simulink model "regionprop_test"  (R2015b)
settings: Solver=VariableStepAuto  StartTime=0.0  StopTime=inf  RelTol=1e-3
PreLoadFcn:
  | coeff = load(coeff_save.mat);
values from neighbouring files (symbols this model uses):
  D = img(max(r2+(c2-1)*sx,1))    [IntegralImage_BoxIntegral_mine.m]
undefined symbols (not defined in the file or in its folder): IsPositionTracked, IsSkeletonTracked, JointDepthIndices, JointImageIndices, JointTrackingState, JointWorldCoordinates, PositionDepthIndices, PositionImageIndices, PositionWorldCoordinates, SegmentationData, SkeletonTrackingID, videoinput
libraries: neural x20, visionsinks x3, visionstatistics x1, imaqlib x1, visionsources x1
(part 1 of 3)
settings Model: Creator=FLM  LastModifiedBy=User

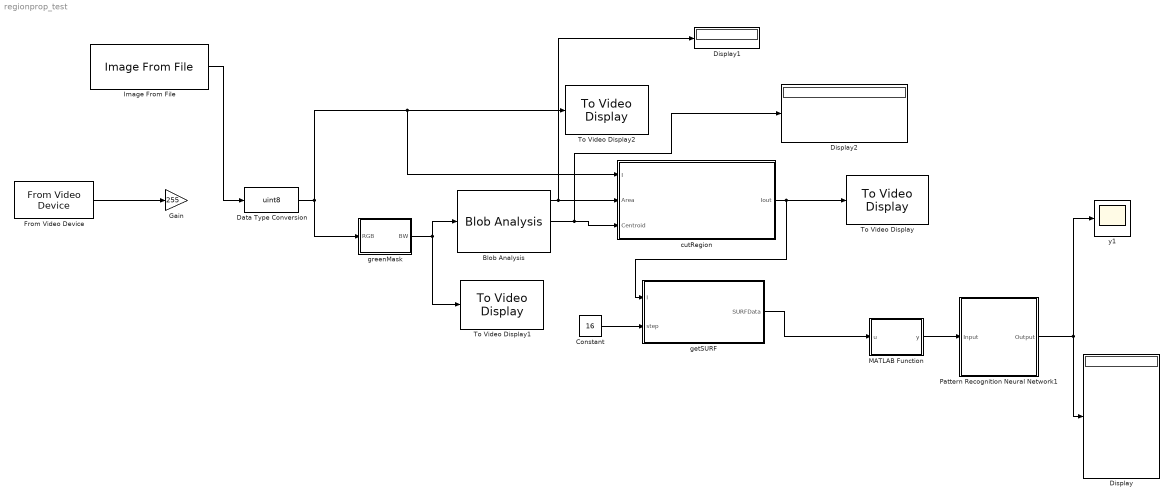
== system regionprop_test ==
  Blob Analysis : visionstatistics/Blob Analysis  Tag=vipblks_row_conv  area=on  centroid=on  bBox=on  majorAxis=off  minorAxis=off  angle=off  eccentricity=off  equivDiameterSq=off  extent=off  perimeter=off  maxBlobs=10  warnIfNumBlobsExceeded=on  isCount=off  useMinArea=off  minArea=0  useMaxArea=off  maxArea=intmax('uint32')  excludeBorderBlob=off  outDT=double  isOutVarDim=off  isFill=on  fillValues=-1  conn=8  isLabel=off  outputMode=Binary point scaling  outputWordLength=32  outputFracLength=16  firstCoeffMode=Binary point scaling  firstCoeffWordLength=16  firstCoeffFracLength=14  secondCoeffMode=Binary point scaling  secondCoeffWordLength=32  secondCoeffFracLength=16  accumMode=Binary point scaling  accumWordLength=32  accumFracLength=0  prodOutputMode=Binary point scaling  prodOutputWordLength=32  prodOutputFracLength=16  roundingMode=Floor  overflowMode=off
  Constant : Constant  Value=16
  Data Type Conversion : DataTypeConversion  OutDataTypeStr=uint8
  Display : Display
  Display1 : Display
  Display2 : Display
  From Video Device : imaqlib/From Video Device  DeviceMenu=winvideo 1 (1.3M HD WebCam)  Device=winvideo 1 (Microsoft? LifeCam Cinema(TM))  ObjConstructor=videoinput('winvideo', 1)  VideoFormatMenu=MJPG_1280x800  VideoFormat=MJPG_320x240  VideoSource=input1  ROIPosition=[0 0 240 320]  EnableHWTrigger=off  TriggerConfiguration=winvideo 1 (1.3M HD WebCam)  SampleTime=1/30  OutputPortsMode=One multidimensional signal  DataType=single  CanDoHWTrigger=no  ReturnedColorSpace=rgb  BlockHandle=1970.0024  ROIWidth=320  ROIHeight=240  ROIColumn=0  ROIRow=0  EngXMLPath=D:\Program Files\MATLAB\R2015b\toolbox\imaq\imaq\private  DevXMLPath=D:\MATLAB\SupportPackages\R2015b\osgenericvideointerface\toolbox\imaq\supportpackages\genericvideo\adaptor\win64  EngLibPath=D:\Program Files\MATLAB\R2015b\toolbox\imaq\imaqblks\imaqmex\win64  ColorSpace=rgb  BayerSensorAlignment=grbg  AllMetadata=IsPositionTracked;IsSkeletonTracked;JointDepthIndices;JointImageIndices;JointTrackingState;JointWorldCoordinates;PositionDepthIndices;PositionImageIndices;PositionWorldCoordinates;SegmentationData;SkeletonTrackingID
  Gain : Gain  Gain=255
  Image From File : visionsources/Image From File  Tag=vipblks_nd  FileName=C:\Users\User\Documents\Ponts 2015-2016\Projet dpt\github\Robot-Sur-Mars\BiggerObjects\Glue\Glue1.png  imagePorts=One multidimensional signal  Ts=inf  ImageDataType=Inherit from input image  Signed=on  WordLength=16  sdImageDataType=uint(8)  FractionLengthMode=User-defined  FractionLength=15  OutPortLabels=R|G|B
  MATLAB Function : MATLAB Function  TreatAsAtomicUnit=on
  Pattern Recognition Neural Network1 : Subsystem
      mask help: Pattern Recognition Neural Network
      mask Display: e = 0.06;c1 = [120 150 230]/255;c2 = ([120 150 230]+0)/383;c3 = ([120 150 230]+128)/383;patch([0 1 1 0],[0 0 1 1],c1);patch([0 1 1 1-e 1-e 0+e],[0 0 1 1-e 0+e 0+e],c2);patch([0 0 1 1-e 0+e 0+e],[0 1 1 1-e 1-e 0+e],c3);plot([0 1 1 0 0],[0 0 1 1 0]);fprintf('NNET');port_label('input',1,' Input');port_label('output',1,'Output ');
  To Video Display : visionsinks/To Video Display  windowSizeMode=Normal  openAtMdlStart=on  fullScreen=off  videoWindowX=1478  videoWindowY=273  saveWindowSize=off  videoWindowWidth=160  videoWindowHeight=160  inputColorFormat=RGB  inputType=Obsolete  imagePorts=One multidimensional signal  OutputDevice=On-screen video monitor  dataOrg=Column-major  isWindowOpen=off
  To Video Display1 : visionsinks/To Video Display  windowSizeMode=Normal  openAtMdlStart=on  fullScreen=off  videoWindowX=839  videoWindowY=303  saveWindowSize=off  videoWindowWidth=160  videoWindowHeight=160  inputColorFormat=RGB  inputType=Obsolete  imagePorts=One multidimensional signal  OutputDevice=On-screen video monitor  dataOrg=Column-major  isWindowOpen=off
  To Video Display2 : visionsinks/To Video Display  windowSizeMode=Normal  openAtMdlStart=on  fullScreen=off  videoWindowX=1504  videoWindowY=564  saveWindowSize=off  videoWindowWidth=160  videoWindowHeight=160  inputColorFormat=RGB  inputType=Obsolete  imagePorts=One multidimensional signal  OutputDevice=On-screen video monitor  dataOrg=Column-major  isWindowOpen=off
  cutRegion : MATLAB Function  TreatAsAtomicUnit=on
  getSURF : MATLAB Function  TreatAsAtomicUnit=on
  greenMask : MATLAB Function  TreatAsAtomicUnit=on
  y1 : Scope
      mask Display: e = 0.06;c1 = [120 230 180]/255;c2 = ([120 230 180]+0)/(256+128);c3 = ([120 230 180]+128)/(256+128);patch([0 1 1 0],[0 0 1 1],c1);patch([0 1 1 1-e 1-e 0+e],[0 0 1 1-e 0+e 0+e],c2);patch([0 0 1 1-e 0+e 0+e],[0 1 1 1-e 1-e 0+e],c3);plot([0 1 1 0 0],[0 0 1 1 0]);plot([0.15 0.85 0.85 0.15 0.15],[0.5 0.5 0.85 0.85 0.5]);
  wires:
  greenMask/1(BW) -> Blob Analysis/1, To Video Display1/1
  Blob Analysis/2 -> Display2/1, cutRegion/3(Centroid)
  Blob Analysis/1 -> cutRegion/2(Area), Display1/1
  Constant/1 -> getSURF/2(step)
  cutRegion/1(Iout) -> To Video Display/1, getSURF/1(I)
  From Video Device/1 -> Gain/1
  Data Type Conversion/1 -> cutRegion/1(I), To Video Display2/1, greenMask/1(RGB)
  getSURF/1(SURFData) -> MATLAB Function/1(u)
  MATLAB Function/1(y) -> Pattern Recognition Neural Network1/1(Input)
  Image From File/1 -> Data Type Conversion/1
  Pattern Recognition Neural Network1/1(Output) -> Display/1, y1/1

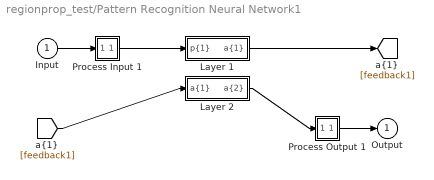
== system regionprop_test/Pattern Recognition Neural Network1 ==
  Input : Inport  PortDimensions=349
      mask Display: e = 0.06;c1 = [120 230 180]/255;c2 = ([120 230 180]+0)/(256+128);c3 = ([120 230 180]+128)/(256+128);patch([0 1 1 0],[0 0 1 1],c1);patch([0 1 1 1-e 1-e 0+e],[0 0 1 1-e 0+e 0+e],c2);patch([0 0 1 1-e 0+e 0+e],[0 1 1 1-e 1-e 0+e],c3);plot([0 1 1 0 0],[0 0 1 1 0]);
  Layer 1 : Subsystem
      mask Display: e = 0.06;c1 = [120 150 230]/255;c2 = ([120 150 230]+0)/383;c3 = ([120 150 230]+128)/383;patch([0 1 1 0],[0 0 1 1],c1);patch([0 1 1 1-e 1-e 0+e],[0 0 1 1-e 0+e 0+e],c2);patch([0 0 1 1-e 0+e 0+e],[0 1 1 1-e 1-e 0+e],c3);plot([0 1 1 0 0],[0 0 1 1 0]);
  Layer 2 : Subsystem
      mask Display: e = 0.06;c1 = [120 150 230]/255;c2 = ([120 150 230]+0)/383;c3 = ([120 150 230]+128)/383;patch([0 1 1 0],[0 0 1 1],c1);patch([0 1 1 1-e 1-e 0+e],[0 0 1 1-e 0+e 0+e],c2);patch([0 0 1 1-e 0+e 0+e],[0 1 1 1-e 1-e 0+e],c3);plot([0 1 1 0 0],[0 0 1 1 0]);
  Process Input 1 : Subsystem
      mask Display: e = 0.06;c1 = [120 150 230]/255;c2 = ([120 150 230]+0)/383;c3 = ([120 150 230]+128)/383;patch([0 1 1 0],[0 0 1 1],c1);patch([0 1 1 1-e 1-e 0+e],[0 0 1 1-e 0+e 0+e],c2);patch([0 0 1 1-e 0+e 0+e],[0 1 1 1-e 1-e 0+e],c3);plot([0 1 1 0 0],[0 0 1 1 0]);
  Process Output 1 : Subsystem
      mask Display: e = 0.06;c1 = [120 150 230]/255;c2 = ([120 150 230]+0)/383;c3 = ([120 150 230]+128)/383;patch([0 1 1 0],[0 0 1 1],c1);patch([0 1 1 1-e 1-e 0+e],[0 0 1 1-e 0+e 0+e],c2);patch([0 0 1 1-e 0+e 0+e],[0 1 1 1-e 1-e 0+e],c3);plot([0 1 1 0 0],[0 0 1 1 0]);
  Output : Outport  InitialOutput=[0;0;0;0;0;0;0]
      mask Display: e = 0.06;c1 = [120 230 180]/255;c2 = ([120 230 180]+0)/(256+128);c3 = ([120 230 180]+128)/(256+128);patch([0 1 1 0],[0 0 1 1],c1);patch([0 1 1 1-e 1-e 0+e],[0 0 1 1-e 0+e 0+e],c2);patch([0 0 1 1-e 0+e 0+e],[0 1 1 1-e 1-e 0+e],c3);plot([0 1 1 0 0],[0 0 1 1 0]);
  wires:
  Input/1 -> Process Input 1/1(x)
  Process Output 1/1(y) -> Output/1
  Process Input 1/1(p) -> Layer 1/1("p{1}")
  Layer 1/1("a{1}") -> [feedback1]
  [feedback1] -> Layer 2/1("a{1} ")
  Layer 2/1("a{2}") -> Process Output 1/1(a)

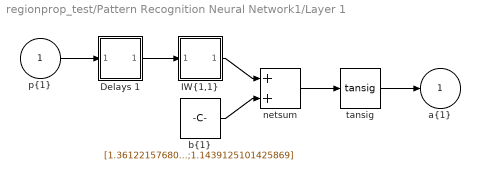
== system regionprop_test/Pattern Recognition Neural Network1/Layer 1 ==
  "p{1}" : Inport  PortDimensions=349
      mask Display: e = 0.06;c1 = [120 230 180]/255;c2 = ([120 230 180]+0)/(256+128);c3 = ([120 230 180]+128)/(256+128);patch([0 1 1 0],[0 0 1 1],c1);patch([0 1 1 1-e 1-e 0+e],[0 0 1 1-e 0+e 0+e],c2);patch([0 0 1 1-e 0+e 0+e],[0 1 1 1-e 1-e 0+e],c3);plot([0 1 1 0 0],[0 0 1 1 0]);
  Delays 1 : Subsystem
      mask Display: e = 0.06;c1 = [120 150 230]/255;c2 = ([120 150 230]+0)/383;c3 = ([120 150 230]+128)/383;patch([0 1 1 0],[0 0 1 1],c1);patch([0 1 1 1-e 1-e 0+e],[0 0 1 1-e 0+e 0+e],c2);patch([0 0 1 1-e 0+e 0+e],[0 1 1 1-e 1-e 0+e],c3);plot([0 1 1 0 0],[0 0 1 1 0]);disp('0');
  "IW{1,1}" : Subsystem
      mask Display: e = 0.06;c1 = [120 150 230]/255;c2 = ([120 150 230]+0)/383;c3 = ([120 150 230]+128)/383;patch([0 1 1 0],[0 0 1 1],c1);patch([0 1 1 1-e 1-e 0+e],[0 0 1 1-e 0+e 0+e],c2);patch([0 0 1 1-e 0+e 0+e],[0 1 1 1-e 1-e 0+e],c3);plot([0 1 1 0 0],[0 0 1 1 0]);disp('W');
  "b{1}" : Constant  Value=[1.3612215768095062;0.94369929257810814;0.60437891866296511;-0.47450873383855663;0.11435504802363132;0.13223426091816515;0.48270888985907545;0.62927800384169408;0.87499647086149779;1.1439125101425869]
      mask Display: e = 0.06;c1 = [120 150 230]/255;c2 = ([120 150 230]+0)/383;c3 = ([120 150 230]+128)/383;patch([0 1 1 0],[0 0 1 1],c1);patch([0 1 1 1-e 1-e 0+e],[0 0 1 1-e 0+e 0+e],c2);patch([0 0 1 1-e 0+e 0+e],[0 1 1 1-e 1-e 0+e],c3);plot([0 1 1 0 0],[0 0 1 1 0]);disp('b');
  netsum : Sum  Inputs=2  SaturateOnIntegerOverflow=on  InputSameDT=on  OutDataTypeStr=Inherit: Same as first input
      mask Display: e = 0.06;c1 = [120 150 230]/255;c2 = ([120 150 230]+0)/383;c3 = ([120 150 230]+128)/383;patch([0 1 1 0],[0 0 1 1],c1);patch([0 1 1 1-e 1-e 0+e],[0 0 1 1-e 0+e 0+e],c2);patch([0 0 1 1-e 0+e 0+e],[0 1 1 1-e 1-e 0+e],c3);plot([0 1 1 0 0],[0 0 1 1 0]);disp('+');
  tansig : neural/Transfer Functions/tansig
  "a{1}" : Outport  InitialOutput=[0;0;0;0;0;0;0;0;0;0]
      mask Display: e = 0.06;c1 = [120 230 180]/255;c2 = ([120 230 180]+0)/(256+128);c3 = ([120 230 180]+128)/(256+128);patch([0 1 1 0],[0 0 1 1],c1);patch([0 1 1 1-e 1-e 0+e],[0 0 1 1-e 0+e 0+e],c2);patch([0 0 1 1-e 0+e 0+e],[0 1 1 1-e 1-e 0+e],c3);plot([0 1 1 0 0],[0 0 1 1 0]);
  wires:
  "p{1}"/1 -> Delays 1/1("p{1}")
  Delays 1/1("pd{1,1}") -> "IW{1,1}"/1("pd{1,1}")
  "IW{1,1}"/1("iz{1,1}") -> netsum/1
  "b{1}"/1 -> netsum/2
  netsum/1 -> tansig/1
  tansig/1 -> "a{1}"/1

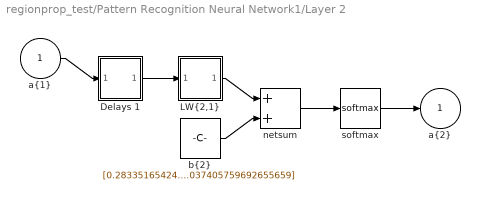
== system regionprop_test/Pattern Recognition Neural Network1/Layer 2 ==
  "a{1} " : Inport  PortDimensions=10
      mask Display: e = 0.06;c1 = [120 230 180]/255;c2 = ([120 230 180]+0)/(256+128);c3 = ([120 230 180]+128)/(256+128);patch([0 1 1 0],[0 0 1 1],c1);patch([0 1 1 1-e 1-e 0+e],[0 0 1 1-e 0+e 0+e],c2);patch([0 0 1 1-e 0+e 0+e],[0 1 1 1-e 1-e 0+e],c3);plot([0 1 1 0 0],[0 0 1 1 0]);
  Delays 1 : Subsystem
      mask Display: e = 0.06;c1 = [120 150 230]/255;c2 = ([120 150 230]+0)/383;c3 = ([120 150 230]+128)/383;patch([0 1 1 0],[0 0 1 1],c1);patch([0 1 1 1-e 1-e 0+e],[0 0 1 1-e 0+e 0+e],c2);patch([0 0 1 1-e 0+e 0+e],[0 1 1 1-e 1-e 0+e],c3);plot([0 1 1 0 0],[0 0 1 1 0]);disp('0');
  "LW{2,1}" : Subsystem
      mask Display: e = 0.06;c1 = [120 150 230]/255;c2 = ([120 150 230]+0)/383;c3 = ([120 150 230]+128)/383;patch([0 1 1 0],[0 0 1 1],c1);patch([0 1 1 1-e 1-e 0+e],[0 0 1 1-e 0+e 0+e],c2);patch([0 0 1 1-e 0+e 0+e],[0 1 1 1-e 1-e 0+e],c3);plot([0 1 1 0 0],[0 0 1 1 0]);disp('W');
  "b{2}" : Constant  Value=[0.28335165424471487;-0.7754437961341617;-0.038493880588752902;-0.37485200974363875;-1.1549457366976141;-0.28396333013774772;0.037405759692655659]
      mask Display: e = 0.06;c1 = [120 150 230]/255;c2 = ([120 150 230]+0)/383;c3 = ([120 150 230]+128)/383;patch([0 1 1 0],[0 0 1 1],c1);patch([0 1 1 1-e 1-e 0+e],[0 0 1 1-e 0+e 0+e],c2);patch([0 0 1 1-e 0+e 0+e],[0 1 1 1-e 1-e 0+e],c3);plot([0 1 1 0 0],[0 0 1 1 0]);disp('b');
  netsum : Sum  Inputs=2  SaturateOnIntegerOverflow=on  InputSameDT=on  OutDataTypeStr=Inherit: Same as first input
      mask Display: e = 0.06;c1 = [120 150 230]/255;c2 = ([120 150 230]+0)/383;c3 = ([120 150 230]+128)/383;patch([0 1 1 0],[0 0 1 1],c1);patch([0 1 1 1-e 1-e 0+e],[0 0 1 1-e 0+e 0+e],c2);patch([0 0 1 1-e 0+e 0+e],[0 1 1 1-e 1-e 0+e],c3);plot([0 1 1 0 0],[0 0 1 1 0]);disp('+');
  softmax : neural/Transfer Functions/softmax
  "a{2}" : Outport  InitialOutput=[0;0;0;0;0;0;0]
      mask Display: e = 0.06;c1 = [120 230 180]/255;c2 = ([120 230 180]+0)/(256+128);c3 = ([120 230 180]+128)/(256+128);patch([0 1 1 0],[0 0 1 1],c1);patch([0 1 1 1-e 1-e 0+e],[0 0 1 1-e 0+e 0+e],c2);patch([0 0 1 1-e 0+e 0+e],[0 1 1 1-e 1-e 0+e],c3);plot([0 1 1 0 0],[0 0 1 1 0]);
  wires:
  "a{1} "/1 -> Delays 1/1("p{2}")
  Delays 1/1("pd{2,1}") -> "LW{2,1}"/1("ad{2,1}")
  "LW{2,1}"/1("lz{2,1}") -> netsum/1
  "b{2}"/1 -> netsum/2
  netsum/1 -> softmax/1
  softmax/1 -> "a{2}"/1

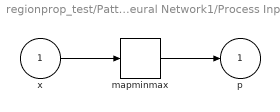
== system regionprop_test/Pattern Recognition Neural Network1/Process Input 1 ==
  x : Inport  PortDimensions=349
      mask Display: e = 0.06;c1 = [120 230 180]/255;c2 = ([120 230 180]+0)/(256+128);c3 = ([120 230 180]+128)/(256+128);patch([0 1 1 0],[0 0 1 1],c1);patch([0 1 1 1-e 1-e 0+e],[0 0 1 1-e 0+e 0+e],c2);patch([0 0 1 1-e 0+e 0+e],[0 1 1 1-e 1-e 0+e],c3);plot([0 1 1 0 0],[0 0 1 1 0]);
  mapminmax : neural/Processing Functions/mapminmax  xmin=[-4185.2254746330764;-3951.2386454701273;-4272.8759210784938;-5275.8951439018438;-4992.6171283589583;-3029.6546894978319;-2069.137827129759;-3698.2789115304699;-1489.2070348176537;-3476.3297599968364;-2650.6012972725089;-2000.8594058807948;-1969.1714593451375;-1789.3272720854163;-1775.7540756503461;-1390.1746543959134;-2206.9243335546894;-1502.6944615907519;-2269.4096947484163;-1388.9568528462191;-1974.9780313183294;-1607.8967104259173;-1209.3166053707982;-1287.1850664751501;-1429.5289070485692;-1354.5409316295572;-1235.0938891011133;-1555.1454403516682;-1179.4053344831818;-1028.9317631149095;-786.01839795641831;-896.33024372702948;-1148.2089370319213;-1354.1679897834128;-1530.573399061785;-906.75073901099552;-813.27565664389249;-1380.3281604440519;-882.57709922812819;-1136.7593180172894;-743.67082005439261;-915.80101255835677;-874.09295999394908;-1285.6890420972377;-751.46533959809017;-1193.6611517563913;-682.55494462015258;-997.29318818897366;-1065.8689820808381;-958.41961059315815;-888.02830061435782;-688.09043680666184;-897.35819316173183;-754.37865037401843;-1005.0606831355447;-915.18687693529102;-762.93745768536644;-918.68258505576978;-677.56257362598672;-902.61100530172075;-624.10096131496186;-615.87677347907402;-658.84660602083363;-720.68385279892436;-562.00862857224547;-741.18599602177869;-621.61961897444462;-691.87562693226243;-663.83944608202523;-626.2452695686452;-568.84176383888382;-855.35400096434694;-503.79560486971695;-838.63228989028607;-554.82755868950085;-649.34461118546938;-602.05003212017209;-731.13156161033078;-603.81023263447378;-627.05373560081739;-642.94809550576042;-644.51257140990651;-507.04200292665757;-551.65208805244458;-411.35195308326115;-493.98579532409508;-518.55699902080846;-538.30424551150986;-487.4750643762307;-389.01542130336429;-775.00539330464233;-528.03042141426749;-486.1254196511963;-651.95596215947239;-448.1069204338778;-407.46295416290417;-616.44815222348382;-489.63561974125071;-444.21354753057756;-516.68443693162033;-522.26968158493116;-432.23901542240026;-367.83667133845256;-436.59037961123238;-488.31381368685493;-469.84682382969959;-590.63427757202271;-359.50288485086804;-416.85318676515158;-433.73293790073814;-552.38744025977894;-444.75448363209466;-445.95203764057607;-359.31725456681556;-519.59646826940207;-434.62867378677299;-434.7676784285743;-592.22417935811745;-459.88760712409749;-374.74808988150153;-447.68074320860779;-321.50062954119562;-407.17416356990873;-329.18351839940738;-642.92312929738614;-330.0108142550323;-289.36375034176956;-336.88026190052301;-434.40346642583188;-392.23173044754435;-339.94787299381971;-466.44952626156748;-434.28027362657258;-472.00195514764988;-312.14556212765035;-338.35092393559739;-405.93728028120927;-361.68307455816705;-340.04774272141026;-273.24472724190628;-324.6396232364628;-336.72069359803061;-346.05915188541394;-268.66682190940855;-257.20330088451442;-328.3115137970251;-282.91746962311242;-427.25624496296786;-363.09739641714935;-361.55365859718677;-339.97833358675314;-351.96930956468441;-317.99889006594776;-354.70088039958773;-410.7797314561281;-277.80200460369161;-368.73685551905055;-386.49949964186391;-308.89046853984837;-445.70186358861946;-310.25016948180496;-387.61439329673851;-237.15844696953997;-303.58747491437902;-271.20937747673634;-326.24170444574861;-353.07974002689139;-341.62448585122672;-291.93592511099291;-273.88822553577916;-360.84189405115734;-251.81206125140406;-261.03041739082568;-360.17243481009314;-285.20019379965493;-236.5920473616103;-294.96328110621982;-362.65109090282351;-222.19672183009305;-313.67236782734557;-394.83138293653695;-275.61707454562816;-224.38876789586587;-329.97670627009336;-303.26608489593184;-258.42693440470555;-285.32685615094556;-279.86355331618336;-263.73901793018734;-281.25418688236232;-280.12055443201888;-308.82714326229086;-271.24942926859404;-256.1063168320602;-254.03201776543887;-267.3224810038331;-245.39706671832519;-277.53308148017277;-239.61455227294189;-235.68225671462724 ...(+2957 chars)]  xmax=[7367.3800706185621;3394.6225376546035;4002.2439674659659;5389.9198345212517;3192.0513182620616;2640.417730937158;3036.2926311315146;1922.9527002381647;2743.4560414538319;2267.9567746343773;2547.7144323611037;2367.9400295458086;1549.1471594771447;1440.7006328692273;1402.6779287952618;1457.2915683364126;1440.1386865120689;2270.6817156868747;1448.6438786643507;1254.3787789941866;1159.1781280480031;1304.3539174091113;1335.9495224870768;1402.45479088305;1576.6263372152885;1139.2250058289342;1662.1264514314155;1252.1541541826327;987.15884193465865;1008.3423920138152;848.38588792095607;1214.0532323299117;1281.1591353947326;824.81902779895108;1318.6070848089989;784.74758153290543;717.10473305528069;1212.326846853703;893.75918895482368;1391.7552106072787;841.66341388602962;862.42327726853944;932.56143174424051;1255.8685117501939;1002.2591665478703;995.72355703196399;908.4225657958491;732.68996320666747;757.96909105802069;798.8113189209115;899.28187053022248;1067.0600048876513;723.04710427215832;783.04396902390818;631.1337449493135;552.21324109255261;1143.2542788184587;1024.0207095165724;598.37868803874187;646.97196368259915;689.50238669021905;665.41177926370642;700.24685346683486;546.35667685319549;766.97229960498805;655.46216725497004;613.65448192502492;714.15686227889671;596.69763948849345;567.27512915336774;574.70448641275004;478.85378396061992;737.99067924706503;521.60253929798819;656.56689134526141;521.85418696822558;562.58644046368408;573.5136660144783;629.43330403099185;614.44428677987287;603.58527386264041;492.95582456207654;696.03824006172044;533.26297506040419;588.95575666347656;499.05724095268192;481.02481003654657;658.22174255871846;526.7355610885287;634.84990287334301;708.63997036721685;603.78856332211603;612.41311498063271;519.64030465753297;476.75378334283471;445.46238590328164;547.00739889618296;503.74285659120619;930.08536766540726;444.7478806664613;576.30538285464866;481.85228995254283;453.54295543380942;430.0854504640339;548.859103850167;563.95909887467542;531.02981004281867;422.97521517374582;401.58688206309159;363.05801753019932;425.48128406180047;459.28008637464728;487.85618188192348;452.7660037526872;345.20335439308951;573.75424851886692;492.13665839890695;376.5829501275133;413.76080601240392;386.71919346304878;345.02219668284374;395.97348247708965;356.35638688764811;366.08656036256275;433.32151328193106;376.75662414090561;440.86316324617218;497.77873679807709;501.68597030806598;298.60093427040317;394.6496043261136;466.30254048311684;333.56546423764718;463.84586143561023;323.23749914546067;358.61233081819813;316.58702849208953;322.43054996385763;395.48020272995211;470.09502435904119;268.00194836055783;335.47550044619044;323.74621165375515;318.89441197906405;350.22215905153473;337.26579205678695;391.82665597114624;301.58735538366358;332.0720414885036;340.7115403683211;400.20370120859275;470.95943314224485;254.06519269579672;516.3307487305824;312.28847583244482;293.14996072488447;362.92573353022226;267.40093290032581;301.61163496969164;313.26428417611646;343.08795801136421;268.07661222563911;260.62300521329962;507.89596199777804;284.82435266260671;306.11312329411476;255.99925427121545;360.64014928919181;284.09612550122665;353.30440737358981;410.3376887730584;376.32906570727039;255.59867040672529;363.54150952291837;280.23635114833075;282.30752757493929;262.73787185681721;303.0786534515002;301.97843428794351;307.69383206731061;259.47852599875819;229.79983530831279;267.65032091475928;267.39303764813064;301.00754773512904;295.92219273229773;328.16423264814421;306.56366478767194;283.27738866849518;303.45693317745031;237.29002696153495;267.97835107005841;312.61793383515425;256.36314263070722;243.51702003313869;278.4089988238303;228.33913390177617;293.8136663751639;273.71830654797964;255.84493192415985;327.90004084767639;300.22980620419185;262.60716642659497;260.90993484439298;365.13767454538583;231.52287106671446;259.19568092729889;245.20644709191023;202.53688006418295;215.94292044155355;300.87925549923534 ...(+2612 chars)]  ymin=-1  ymax=1
  p : Outport  PortDimensions=349
      mask Display: e = 0.06;c1 = [120 230 180]/255;c2 = ([120 230 180]+0)/(256+128);c3 = ([120 230 180]+128)/(256+128);patch([0 1 1 0],[0 0 1 1],c1);patch([0 1 1 1-e 1-e 0+e],[0 0 1 1-e 0+e 0+e],c2);patch([0 0 1 1-e 0+e 0+e],[0 1 1 1-e 1-e 0+e],c3);plot([0 1 1 0 0],[0 0 1 1 0]);
  wires:
  x/1 -> mapminmax/1
  mapminmax/1 -> p/1

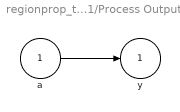
== system regionprop_test/Pattern Recognition Neural Network1/Process Output 1 ==
  a : Inport  PortDimensions=7
      mask Display: e = 0.06;c1 = [120 230 180]/255;c2 = ([120 230 180]+0)/(256+128);c3 = ([120 230 180]+128)/(256+128);patch([0 1 1 0],[0 0 1 1],c1);patch([0 1 1 1-e 1-e 0+e],[0 0 1 1-e 0+e 0+e],c2);patch([0 0 1 1-e 0+e 0+e],[0 1 1 1-e 1-e 0+e],c3);plot([0 1 1 0 0],[0 0 1 1 0]);
  y : Outport  PortDimensions=7
      mask Display: e = 0.06;c1 = [120 230 180]/255;c2 = ([120 230 180]+0)/(256+128);c3 = ([120 230 180]+128)/(256+128);patch([0 1 1 0],[0 0 1 1],c1);patch([0 1 1 1-e 1-e 0+e],[0 0 1 1-e 0+e 0+e],c2);patch([0 0 1 1-e 0+e 0+e],[0 1 1 1-e 1-e 0+e],c3);plot([0 1 1 0 0],[0 0 1 1 0]);
  wires:
  a/1 -> y/1

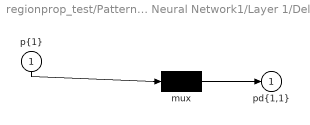
== system regionprop_test/Pattern Recognition Neural Network1/Layer 1/Delays 1 ==
  "p{1}" : Inport  PortDimensions=349
      mask Display: e = 0.06;c1 = [120 230 180]/255;c2 = ([120 230 180]+0)/(256+128);c3 = ([120 230 180]+128)/(256+128);patch([0 1 1 0],[0 0 1 1],c1);patch([0 1 1 1-e 1-e 0+e],[0 0 1 1-e 0+e 0+e],c2);patch([0 0 1 1-e 0+e 0+e],[0 1 1 1-e 1-e 0+e],c3);plot([0 1 1 0 0],[0 0 1 1 0]);
  mux : Mux  Inputs=1
      mask Display: e = 0.06;c1 = [120 150 230]/255;c2 = ([120 150 230]+0)/383;c3 = ([120 150 230]+128)/383;patch([0 1 1 0],[0 0 1 1],c1);patch([0 1 1 1-e 1-e 0+e],[0 0 1 1-e 0+e 0+e],c2);patch([0 0 1 1-e 0+e 0+e],[0 1 1 1-e 1-e 0+e],c3);plot([0 1 1 0 0],[0 0 1 1 0]);disp('Mux')
  "pd{1,1}" : Outport
      mask Display: e = 0.06;c1 = [120 230 180]/255;c2 = ([120 230 180]+0)/(256+128);c3 = ([120 230 180]+128)/(256+128);patch([0 1 1 0],[0 0 1 1],c1);patch([0 1 1 1-e 1-e 0+e],[0 0 1 1-e 0+e 0+e],c2);patch([0 0 1 1-e 0+e 0+e],[0 1 1 1-e 1-e 0+e],c3);plot([0 1 1 0 0],[0 0 1 1 0]);
  wires:
  "p{1}"/1 -> mux/1
  mux/1 -> "pd{1,1}"/1
